simulink model "test"  (R2014b)
settings: Solver=ode45  SolverMode=SingleTasking  StartTime=0.0  StopTime=10.0  MaxStep=0.01  RelTol=1e-3
values from neighbouring files (symbols this model uses):
  A = eval(As)    [fourinputslq_and_yaw_rate_control.m]
  B = eval(Bs)    [fourinputslq_and_yaw_rate_control.m]
  Cs = [1 0 0 0 0 0; 0 1 0 0 0 0; 0 0 1 0 0 0;  0 0 0 1 0 0;0 0 0 0 1 0]    [fourinputslq_and_yaw_rate_control.m]
undefined symbols (not defined in the file or in its folder): K
settings Model: CovSFcnEnable=on  Creator=Jaby  LastModifiedBy=danielpihlquist
settings OptimizationCC: BlockReduction=off  BooleanDataType=off  UseDivisionForNetSlopeComputation=off  SimCompilerOptimization=off
settings DebuggingCC: SaveWithParameterizedLinksMsg=none  UnderspecifiedInitializationDetection=Classic  MergeDetectMultiDrivingBlocksExec=none  SignalResolutionControl=TryResolveAllWithWarning  SolverPrmCheckMsg=none  FrameProcessingCompatibilityMsg=error
settings HardwareCC: TargetUnknown=on
settings RTWCC: RTWCompilerOptimization=off

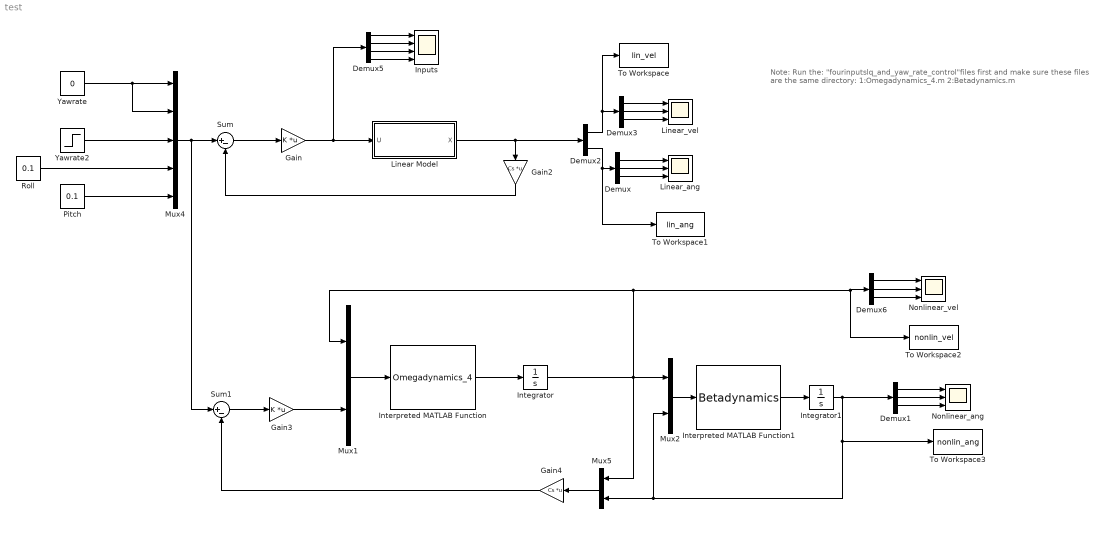
== system test ==
  note: Note:
      | Run the: "fourinputslq_and_yaw_rate_control"files first and make sure these files are the same directory:
      | 1:Omegadynamics_4.m
      | 2:Betadynamics.m
  Demux{,1,3,6} (4 alike) : Demux  Outputs=3
  Demux2 : Demux  Outputs=2
  Demux5 : Demux
  Gain : Gain  Gain=K  Multiplication=Matrix(K*u)
  Gain2 : Gain  Gain=Cs  Multiplication=Matrix(K*u)
  Gain3 : Gain  Gain=K  Multiplication=Matrix(K*u)
  Gain4 : Gain  Gain=Cs  Multiplication=Matrix(K*u)
  Inputs : Scope  NumInputPorts=4
      settings: TimeRange=20  YMin=0.00274~-3.07e-14~8.3e-31~-5  YMax=0.00278~-3.025e-14~8.43e-31~5  SaveName=ScopeData4
  Integrator : Integrator  InitialCondition=[0 0 0]'
  Integrator1 : Integrator  InitialCondition=[0 0 0]'
  Interpreted MATLAB Function : MATLABFcn  MATLABFcn=Omegadynamics_4  Output1D=off
  Interpreted MATLAB Function1 : MATLABFcn  MATLABFcn=Betadynamics  Output1D=off
  "Linear Model " : Subsystem
  Linear_ang : Scope  NumInputPorts=3
      settings: TimeRange=20  YMin=0.00274~-3.07e-14~8.3e-31  YMax=0.00278~-3.025e-14~8.43e-31
  Linear_vel : Scope  NumInputPorts=3
      settings: TimeRange=10  YMin=-6e-17~-0.09~0.97  YMax=2e-17~0.01~1  SaveName=ScopeData2
  Mux1 : Mux  Inputs=2
  Mux2 : Mux  Inputs=2
  Mux4 : Mux  Inputs=5
  Mux5 : Mux  Inputs=2
  Nonlinear_ang : Scope  NumInputPorts=3
      settings: TimeRange=20  YMin=0.00274~-3.07e-14~8.3e-31  YMax=0.00278~-3.025e-14~8.43e-31
  Nonlinear_vel : Scope  NumInputPorts=3
      settings: TimeRange=10  YMin=0~-0.5~-400000  YMax=2.5~2~0  SaveName=ScopeData5
  Pitch : Constant  Value=0.1
  Roll : Constant  Value=0.1
  Sum : Sum  Inputs=|+-
  Sum1 : Sum  Inputs=|+-
  To Workspace : ToWorkspace  VariableName=lin_vel  SampleTime=-1
  To Workspace1 : ToWorkspace  VariableName=lin_ang  SampleTime=-1
  To Workspace2 : ToWorkspace  VariableName=nonlin_vel  SampleTime=-1
  To Workspace3 : ToWorkspace  VariableName=nonlin_ang  SampleTime=-1
  Yawrate : Constant  Value=0
  Yawrate2 : Step  Time=5  After=0.1  SampleTime=0
  wires:
  Demux/1 -> Linear_ang/1
  Demux/2 -> Linear_ang/2
  Demux/3 -> Linear_ang/3
  Integrator/1 -> To Workspace2/1, Demux6/1, Mux1/1, Mux2/1, Mux5/1
  Mux1/1 -> Interpreted MATLAB Function/1
  Interpreted MATLAB Function/1 -> Integrator/1
  Interpreted MATLAB Function1/1 -> Integrator1/1
  Demux2/2 -> To Workspace1/1, Demux/1
  Demux3/1 -> Linear_vel/1
  Demux3/2 -> Linear_vel/2
  Demux3/3 -> Linear_vel/3
  "Linear Model "/1(X) -> Demux2/1, Gain2/1
  Demux5/1 -> Inputs/1
  Demux5/2 -> Inputs/2
  Demux5/3 -> Inputs/3
  Mux5/1 -> Gain4/1
  Mux2/1 -> Interpreted MATLAB Function1/1
  Demux2/1 -> Demux3/1, To Workspace/1
  Demux1/1 -> Nonlinear_ang/1
  Demux1/2 -> Nonlinear_ang/2
  Demux1/3 -> Nonlinear_ang/3
  Integrator1/1 -> Demux1/1, To Workspace3/1, Mux2/2, Mux5/2
  Demux6/1 -> Nonlinear_vel/1
  Demux6/2 -> Nonlinear_vel/2
  Demux6/3 -> Nonlinear_vel/3
  Demux5/4 -> Inputs/4
  Gain2/1 -> Sum/2
  Sum/1 -> Gain/1
  Gain/1 -> Demux5/1, "Linear Model "/1(U)
  Mux4/1 -> Sum1/1, Sum/1
  Roll/1 -> Mux4/4
  Yawrate2/1 -> Mux4/3
  Pitch/1 -> Mux4/5
  Yawrate/1 -> Mux4/2, Mux4/1
  Sum1/1 -> Gain3/1
  Gain3/1 -> Mux1/2
  Gain4/1 -> Sum1/2

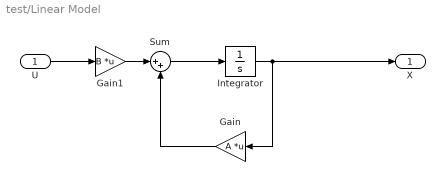
== system test/Linear Model  ==
  U : Inport
  Gain : Gain  Gain=A  Multiplication=Matrix(K*u)
  Gain1 : Gain  Gain=B  Multiplication=Matrix(K*u)
  Integrator : Integrator
  Sum : Sum  Inputs=|++
  X : Outport
  wires:
  Integrator/1 -> X/1, Gain/1
  U/1 -> Gain1/1
  Gain1/1 -> Sum/1
  Sum/1 -> Integrator/1
  Gain/1 -> Sum/2
